simulink model "xy_compare"  (R2018a)
settings: Solver=VariableStepAuto  StartTime=0.0  StopTime=20  RelTol=1e-3
undefined symbols (not defined in the file): drone, est_c_A, est_c_B, est_c_C, est_c_D, regulator_gain_of_attitude, simulation_sampling_ts
libraries: simulink x1
settings Model: Creator=ros  LastModifiedBy=ros

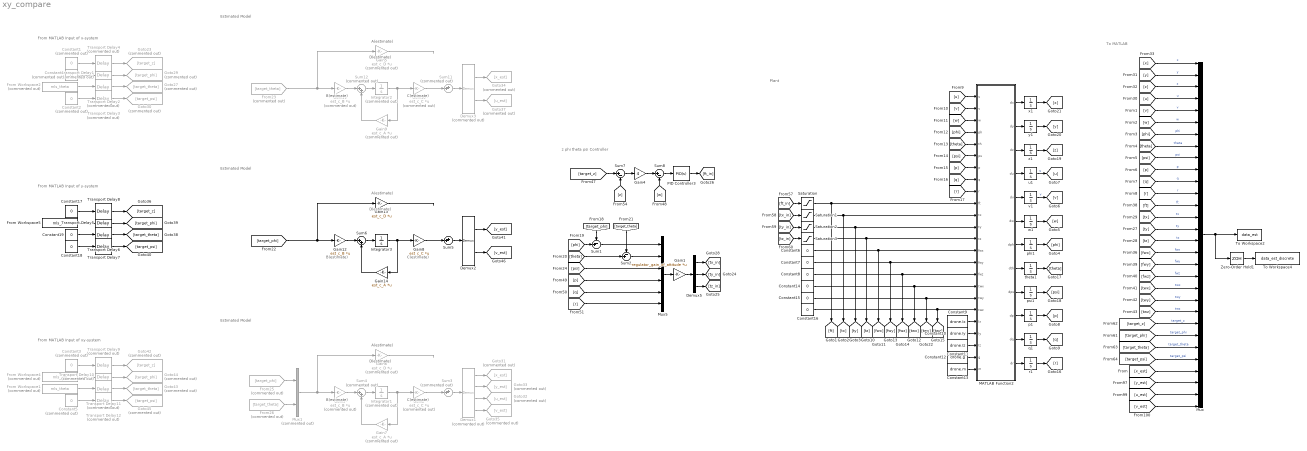
== system xy_compare ==
  note: To MATLAB
  note: Estimated Model
  note: A(estimate)
  note: B(estimate)
  note: C(estimate)
  note: D(estimate)
  note: z phi theta psi Controller
  note: Plant
  note: D(estimate)
  note: A(estimate)
  note: B(estimate)
  note: Estimated Model
  note: C(estimate)
  note: From MATLAB Input of xy-system
  note: From MATLAB Input of x-system
  note: A(estimate)
  note: B(estimate)
  note: Estimated Model
  note: D(estimate)
  note: C(estimate)
  note: From MATLAB Input of y-system
  Constant{1..5} (5 alike) : Constant  Commented=on  Value=0
  Constant10 : Constant  Value=drone.Iy
  Constant11 : Constant  Value=drone.Iz
  Constant12 : Constant  Value=drone.g
  Constant13 : Constant  Value=drone.m
  Constant{6..8,14..19} (9 alike) : Constant  Value=0
  Constant9 : Constant  Value=drone.Ix
  Demux1 : Demux  Commented=on
  Demux2 : Demux  Outputs=2
  Demux3 : Demux  Commented=on  Outputs=2
  Demux5 : Demux  Outputs=3
  From Workspace1 : FromWorkspace  Commented=on  VariableName=mls_theta  SampleTime=0
  From Workspace2 : FromWorkspace  Commented=on  VariableName=mls_theta  SampleTime=0
  From Workspace4 : FromWorkspace  Commented=on  VariableName=mls_phi  SampleTime=0
  From Workspace5 : FromWorkspace  VariableName=mls_phi  SampleTime=0
  From23 : From  Commented=on  GotoTag=target_theta
  From25 : From  Commented=on  GotoTag=target_phi
  From26 : From  Commented=on  GotoTag=target_theta
  Gain1 : Gain  Gain=-regulator_gain_of_attitude  Multiplication=Matrix(K*u)
  Gain10 : Gain  Commented=on  Gain=est_c_C  Multiplication=Matrix(K*u)
  Gain11 : Gain  Commented=on  Gain=est_c_B  Multiplication=Matrix(K*u)
  Gain12 : Gain  Gain=est_c_B  Multiplication=Matrix(K*u)
  Gain13 : Gain  Gain=est_c_D  Multiplication=Matrix(K*u)
  Gain14 : Gain  Gain=est_c_A  Multiplication=Matrix(K*u)
  Gain2 : Gain  Commented=on  Gain=est_c_C  Multiplication=Matrix(K*u)
  Gain3 : Gain  Commented=on  Gain=est_c_B  Multiplication=Matrix(K*u)
  Gain4 : Gain  Gain=4
  Gain5 : Gain  Commented=on  Gain=est_c_D  Multiplication=Matrix(K*u)
  Gain6 : Gain  Commented=on  Gain=est_c_D  Multiplication=Matrix(K*u)
  Gain7 : Gain  Commented=on  Gain=est_c_A  Multiplication=Matrix(K*u)
  Gain8 : Gain  Gain=est_c_C  Multiplication=Matrix(K*u)
  Gain9 : Gain  Commented=on  Gain=est_c_A  Multiplication=Matrix(K*u)
  Goto23 : Goto  Commented=on  GotoTag=target_z
  Goto27 : Goto  Commented=on  GotoTag=target_theta
  Goto29 : Goto  Commented=on  GotoTag=target_phi
  Goto30 : Goto  Commented=on  GotoTag=target_psi
  Goto31 : Goto  Commented=on  GotoTag=x_est
  Goto32 : Goto  Commented=on  GotoTag=u_est
  Goto33 : Goto  Commented=on  GotoTag=y_est
  Goto34 : Goto  Commented=on  GotoTag=x_est
  Goto35 : Goto  Commented=on  GotoTag=v_est
  Goto37 : Goto  Commented=on  GotoTag=u_est
  Goto42 : Goto  Commented=on  GotoTag=target_z
  Goto43 : Goto  Commented=on  GotoTag=target_theta
  Goto44 : Goto  Commented=on  GotoTag=target_phi
  Goto45 : Goto  Commented=on  GotoTag=target_psi
  Integrator1 : Integrator  Commented=on
  Integrator2 : Integrator  Commented=on
  Integrator3 : Integrator
  MATLAB Function2 : MATLAB Function  TreatAsAtomicUnit=on
  Mux : Mux  Inputs=30
  Mux1 : Mux  Commented=on  Inputs=2
  Mux5 : Mux  Inputs=6
  PID Controller3 : simulink/Continuous/PID Controller  Controller=PID  TimeDomain=Continuous-time  SampleTime=-1  IntegratorMethod=Forward Euler  FilterMethod=Forward Euler  Form=Parallel  UseFilter=on  ControllerParametersSource=internal  P=7  I=6  D=0.7  N=100  InitialConditionSource=internal  InitialConditionForIntegrator=0  InitialConditionForFilter=0  ExternalReset=none  LimitOutput=off  UpperSaturationLimit=inf  LowerSaturationLimit=-inf  LinearizeAsGain=on  AntiWindupMode=none  Kb=1  TrackingMode=off  Kt=1  PParamMin=[]  PParamMax=[]  IParamMin=[]  IParamMax=[]  DParamMin=[]  DParamMax=[]  NParamMin=[]  NParamMax=[]  KbParamMin=[]  KbParamMax=[]  KtParamMin=[]  KtParamMax=[]  POutMin=[]  POutMax=[]  IOutMin=[]  IOutMax=[]  DOutMin=[]  DOutMax=[]  NOutMin=[]  NOutMax=[]  KbOutMin=[]  KbOutMax=[]  KtOutMin=[]  KtOutMax=[]  IntegratorOutMin=[]  IntegratorOutMax=[]  FilterOutMin=[]  FilterOutMax=[]  SumOutMin=[]  SumOutMax=[]  SumI1OutMin=[]  SumI1OutMax=[]  SumI2OutMin=[]  SumI2OutMax=[]  SumI3OutMin=[]  SumI3OutMax=[]  SumDOutMin=[]  SumDOutMax=[]  SaturationOutMin=[]  SaturationOutMax=[]  IntegratorContinuousStateAttributes=''  IntegratorStateMustResolveToSignalObject=off  IntegratorRTWStateStorageClass=Auto  FilterContinuousStateAttributes=''  FilterStateMustResolveToSignalObject=off  FilterRTWStateStorageClass=Auto  DifferentiatorICPrevScaledInput=0  DifferentiatorOutMin=[]  DifferentiatorOutMax=[]  FilterDiffOutCoefMin=[]  FilterDiffOutCoefMax=[]  SumDenOutMin=[]  SumDenOutMax=[]  SumNumOutMin=[]  SumNumOutMax=[]  ReciprocalOutMin=[]  ReciprocalOutMax=[]  DivideOutMin=[]  DivideOutMax=[]  TunerSelectOption=Transfer Function Based (PID Tuner App)
  Saturation{,1..3} (4 alike) : Saturate  UpperLimit=30  LowerLimit=-100
  Sum1 : Sum  Inputs=-+|
  Sum11 : Sum  Commented=on  Inputs=++|
  Sum12 : Sum  Commented=on  Inputs=|++
  Sum2 : Sum  Inputs=-+|
  Sum3 : Sum  Commented=on  Inputs=++|
  Sum4 : Sum  Commented=on  Inputs=|++
  Sum5 : Sum  Inputs=++|
  Sum6 : Sum  Inputs=|++
  Sum7 : Sum  Inputs=|+-
  Sum8 : Sum  Inputs=|+-
  To Workspace2 : ToWorkspace  VariableName=data_est  SaveFormat=Timeseries  SampleTime=-1
  To Workspace4 : ToWorkspace  VariableName=data_est_discrete  SaveFormat=Timeseries  SampleTime=-1
  Transport Delay{1..4,9..12} (8 alike) : TransportDelay  Commented=on  DelayTime=10
  Transport Delay{5..8} (4 alike) : TransportDelay  DelayTime=10
  Zero-Order Hold1 : ZeroOrderHold  SampleTime=simulation_sampling_ts
  p1 : Integrator
  phi1 : Integrator
  psi1 : Integrator
  q1 : Integrator
  r1 : Integrator
  theta1 : Integrator
  u1 : Integrator
  v1 : Integrator
  w1 : Integrator
  x1 : Integrator
  y1 : Integrator
  z1 : Integrator
  wires:
  [x] -> Mux/1  "x"
  [v] -> Mux/5  "v"
  [z] -> Mux/3  "z"
  [w] -> Mux/6  "w"
  [p] -> Mux/10  "p"
  [phi] -> Mux/7  "phi"
  [theta] -> Mux/8  "theta"
  [r] -> Mux/12  "r"
  [y] -> Mux/2  "y"
  [psi] -> Mux/9  "psi"
  [u] -> Mux/4  "u"
  [q] -> Mux/11  "q"
  Mux/1 -> Zero-Order Hold1/1, To Workspace2/1
  [ft] -> Mux/13  "ft"
  [tx] -> Mux/14  "tx"
  [ty] -> Mux/15  "ty"
  [tz] -> Mux/16  "tz"
  [fwx] -> Mux/17  "fwx"
  [fwy] -> Mux/18  "fwy"
  [fwz] -> Mux/19  "fwz"
  [twx] -> Mux/20  "twx"
  [twy] -> Mux/21  "twy"
  [twz] -> Mux/22  "twz"
  Zero-Order Hold1/1 -> To Workspace4/1
  [target_z] -> Mux/23  "target_z"
  [target_phi] -> Mux/24  "target_phi"
  [target_theta] -> Mux/25  "target_theta"
  [target_psi] -> Mux/26  "target_psi"
  [x_est] -> Mux/27
  [y_est] -> Mux/28
  Demux3/1 -> Goto34/1
  Sum11/1 -> Demux3/1
  Integrator2/1 -> Gain10/1, Gain9/1
  Gain5/1 -> ?
  Gain11/1 -> Sum12/1
  Gain9/1 -> Sum12/2
  Gain10/1 -> Sum11/2
  Sum12/1 -> Integrator2/1
  From23/1 -> Gain5/1, Gain11/1
  Demux3/2 -> Goto37/1
  PID Controller3/1 -> [ft_in]
  [target_z] -> Sum7/1
  Sum1/1 -> Mux5/1
  Sum2/1 -> Mux5/2
  [theta] -> Sum2/2
  Demux5/3 -> [tz_in]
  Sum8/1 -> PID Controller3/1
  [z] -> Sum7/2
  Demux5/2 -> [ty_in]
  [r] -> Mux5/6
  [q] -> Mux5/5
  Demux5/1 -> [tx_in]
  [phi] -> Sum1/2
  [target_theta] -> Sum2/1
  Gain1/1 -> Demux5/1
  Sum7/1 -> Gain4/1
  [target_phi] -> Sum1/1
  [w] -> Sum8/2
  Mux5/1 -> Gain1/1
  [psi] -> Mux5/3
  [p] -> Mux5/4
  Gain4/1 -> Sum8/1
  v1/1 -> [v]  "v"
  MATLAB Function2/8(dth) -> theta1/1
  [ft_in] -> Saturation/1
  MATLAB Function2/10(dp) -> p1/1
  Constant16/1 -> [twz], MATLAB Function2/19(twz)
  MATLAB Function2/12(dr) -> r1/1
  MATLAB Function2/2(dy) -> y1/1
  Constant8/1 -> [fwz], MATLAB Function2/16(fwz)
  w1/1 -> [w]
  MATLAB Function2/4(du) -> u1/1
  phi1/1 -> [phi]
  Constant15/1 -> [twy], MATLAB Function2/18(twy)
  [q] -> MATLAB Function2/8(q)
  [tz_in] -> Saturation3/1
  MATLAB Function2/7(dph) -> phi1/1
  Constant6/1 -> [fwx], MATLAB Function2/14(fwx)
  Saturation/1 -> [ft], MATLAB Function2/10(ft)
  Saturation3/1 -> [tz], MATLAB Function2/13(tz)
  [phi] -> MATLAB Function2/4(ph)
  Constant13/1 -> MATLAB Function2/24(m)
  Constant9/1 -> MATLAB Function2/20(Ix)
  z1/1 -> [z]
  q1/1 -> [q]
  psi1/1 -> [psi]
  [r] -> MATLAB Function2/9(r)
  [theta] -> MATLAB Function2/5(th)
  MATLAB Function2/5(dv) -> v1/1
  Constant12/1 -> MATLAB Function2/23(g)
  Saturation2/1 -> [ty], MATLAB Function2/12(ty)
  r1/1 -> [r]
  Constant7/1 -> [fwy], MATLAB Function2/15(fwy)
  MATLAB Function2/9(dps) -> psi1/1
  Constant11/1 -> MATLAB Function2/22(Iz)
  [p] -> MATLAB Function2/7(p)
  theta1/1 -> [theta]
  [psi] -> MATLAB Function2/6(ps)
  x1/1 -> [x]
  MATLAB Function2/3(dz) -> z1/1
  [ty_in] -> Saturation2/1
  Constant10/1 -> MATLAB Function2/21(Iy)
  MATLAB Function2/11(dq) -> q1/1
  y1/1 -> [y]
  [w] -> MATLAB Function2/3(w)
  [u] -> MATLAB Function2/1(u)
  [v] -> MATLAB Function2/2(v)
  MATLAB Function2/6(dw) -> w1/1
  u1/1 -> [u]  "u"
  p1/1 -> [p]
  Saturation1/1 -> [tx], MATLAB Function2/11(tx)
  Constant14/1 -> [twx], MATLAB Function2/17(twx)
  MATLAB Function2/1(dx) -> x1/1
  [tx_in] -> Saturation1/1
  [v_est] -> Mux/30
  [u_est] -> Mux/29
  Integrator1/1 -> Gain2/1, Gain7/1
  Gain6/1 -> ?
  Demux1/1 -> Goto31/1
  Demux1/2 -> Goto33/1
  Demux1/3 -> Goto32/1
  From26/1 -> Mux1/2
  Mux1/1 -> Gain6/1, Gain3/1
  Demux1/4 -> Goto35/1
  From25/1 -> Mux1/1
  Gain2/1 -> Sum3/2
  Sum3/1 -> Demux1/1
  Sum4/1 -> Integrator1/1
  Gain3/1 -> Sum4/1
  Gain7/1 -> Sum4/2
  Constant5/1 -> Transport Delay12/1
  Constant1/1 -> Transport Delay4/1
  From Workspace1/1 -> Transport Delay11/1
  Transport Delay2/1 -> Goto27/1
  Transport Delay4/1 -> Goto23/1
  From Workspace2/1 -> Transport Delay2/1
  Transport Delay10/1 -> Goto44/1
  Transport Delay3/1 -> Goto30/1
  Constant4/1 -> Transport Delay1/1
  Transport Delay11/1 -> Goto43/1
  Transport Delay1/1 -> Goto29/1
  Transport Delay9/1 -> Goto42/1
  Constant3/1 -> Transport Delay9/1
  Constant2/1 -> Transport Delay3/1
  From Workspace4/1 -> Transport Delay10/1
  Transport Delay12/1 -> Goto45/1
  Gain13/1 -> ?
  Demux2/1 -> [y_est]
  [target_phi] -> Gain13/1, Gain12/1
  Gain8/1 -> Sum5/2
  Integrator3/1 -> Gain8/1, Gain14/1
  Demux2/2 -> [v_est]
  Sum5/1 -> Demux2/1
  Sum6/1 -> Integrator3/1
  Gain12/1 -> Sum6/1
  Gain14/1 -> Sum6/2
  Constant18/1 -> Transport Delay7/1
  Transport Delay7/1 -> [target_psi]
  Constant19/1 -> Transport Delay6/1
  Transport Delay8/1 -> [target_z]
  Transport Delay5/1 -> [target_phi]
  Transport Delay6/1 -> [target_theta]
  Constant17/1 -> Transport Delay8/1
  From Workspace5/1 -> Transport Delay5/1

== matlab function xy_compare/MATLAB Function2 ==
  data: u input; v input; dx output; w input; ph input; th input; ps input; p input; q input; r input; ft input; tx input; ty input; tz input; fwx input; fwy input; fwz input; twx input; twy input; twz input; dy output; dz output; du output; dv output; dw output; dph output; dth output; dps output; dp output; dq output; dr output; Ix input; Iy input; Iz input; g input; m input
function [dx, dy, dz, du, dv, dw, dph, dth, dps, dp, dq, dr] = fcn(u, v, w, ph, th, ps, p, q, r, ft, tx, ty, tz, fwx, fwy, fwz, twx, twy, twz, Ix, Iy, Iz, g, m)

dx = w*(sin(ph)*sin(ps) + cos(ph)*cos(ps)*sin(th)) - v*(cos(ph)*sin(ps) - cos(ps)*sin(ph)*sin(th)) + u*(cos(ps)*cos(th));
dy = v*(cos(ph)*cos(ps) + sin(ph)*sin(ps)*sin(th)) - w*(cos(ps)*sin(ph) - cos(ph)*sin(ps)*sin(th)) + u*(cos(th)*sin(ps));
dz = w*(cos(ph)*cos(th)) - u*(sin(th)) + v*(cos(th)*sin(ph));
du = r*v - q*w + g*(sin(th)) + fwx / m;
dv = p*w - r*u - g*(sin(ph)*cos(th)) + fwy / m;
dw = q*u - p*v - g*(cos(th)*cos(ph)) + (fwz + ft) / m;
dph = p + r*(cos(ph)*tan(th)) + q*(sin(ph)*tan(th));
dth = q*(cos(th)) - r*(sin(ph));
dps = r*(cos(ph)/cos(th)) + q*(sin(ph)/cos(th));
dp = r*q*(Iy - Iz)/Ix + (tx + twx)/Ix;
dq = p*r*(Iz - Ix)/Iy + (ty + twy)/Iy;
dr = p*q*(Ix - Iy)/Iz + (tz + twz)/Iz;
